simulink model "calcul_vitesse_roues"  (R2024b)
settings: Solver=FixedStepDiscrete  StartTime=0.0  StopTime=10.0  FixedStep=Ts  RelTol=1e-3
values from neighbouring files (symbols this model uses):
  J = 0.5    [main_data_vehicle.m]
  Re = 0.228    [main_data_vehicle.m]
  v0 = 0.1    [main_data_vehicle.m]
undefined symbols (not defined in the file or in its folder): DiscIntNeverNeededParam
settings Model: Creator=marti  LastModifiedBy=marti

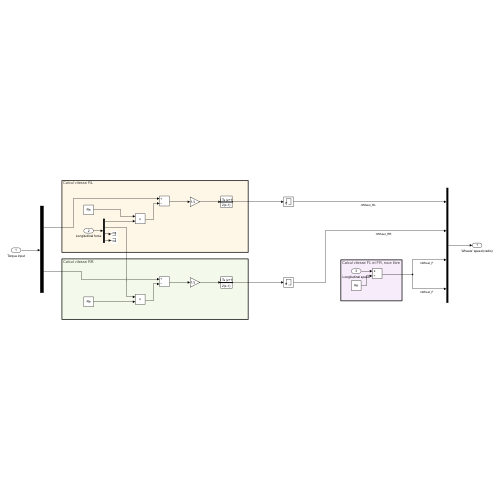
[thumbnail: Simulink's stored preview of the top-level diagram]
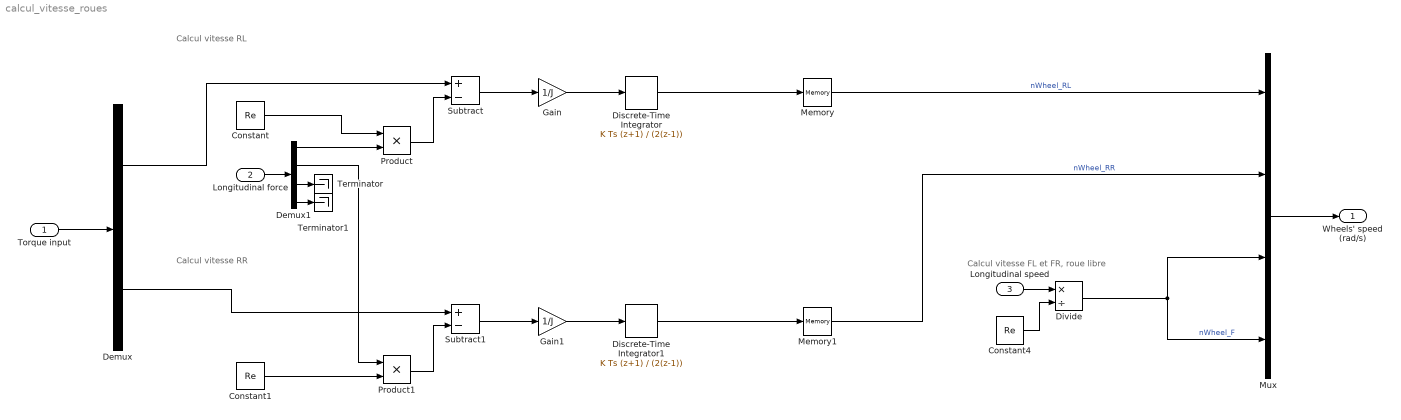
== system calcul_vitesse_roues ==
  note: Calcul vitesse FL et FR, roue libre
  note: Calcul vitesse RL
  note: Calcul vitesse RR
  Torque input : Inport
  Longitudinal force : Inport  Port=2
  Longitudinal speed : Inport  Port=3
  Constant : Constant  Value=Re
  Constant1 : Constant  Value=Re
  Constant4 : Constant  Value=Re
  Demux : Demux  Outputs=2
  Demux1 : Demux
  Discrete-Time Integrator : DiscreteIntegrator  IntegratorMethod=Integration: Trapezoidal  InitialCondition=v0/Re  SampleTime=-1  ICPrevOutput=DiscIntNeverNeededParam  ICPrevScaledInput=DiscIntNeverNeededParam
  Discrete-Time Integrator1 : DiscreteIntegrator  IntegratorMethod=Integration: Trapezoidal  InitialCondition=v0/Re  SampleTime=-1  ICPrevOutput=DiscIntNeverNeededParam  ICPrevScaledInput=DiscIntNeverNeededParam
  Divide : Product  Inputs=*/
  Gain : Gain  Gain=1/J
  Gain1 : Gain  Gain=1/J
  Memory : Memory  InitialCondition=v0/Re
  Memory1 : Memory  InitialCondition=v0/Re
  Mux : Mux
  Product : Product
  Product1 : Product
  Subtract : Sum  Inputs=+-
  Subtract1 : Sum  Inputs=+-
  Terminator : Terminator
  Terminator1 : Terminator
  Wheels' speed (rad/s) : Outport
  wires:
  Product/1 -> Subtract/2
  Subtract/1 -> Gain/1
  Torque input/1 -> Demux/1
  Demux/1 -> Subtract/1
  Longitudinal speed/1 -> Divide/1
  Constant4/1 -> Divide/2
  Mux/1 -> Wheels' speed (rad/s)/1
  Longitudinal force/1 -> Demux1/1
  Demux1/1 -> Product/2
  Constant/1 -> Product/1
  Gain/1 -> Discrete-Time Integrator/1
  Product1/1 -> Subtract1/2
  Gain1/1 -> Discrete-Time Integrator1/1
  Subtract1/1 -> Gain1/1
  Constant1/1 -> Product1/2
  Demux1/2 -> Product1/1
  Demux/2 -> Subtract1/1
  Demux1/3 -> Terminator/1
  Demux1/4 -> Terminator1/1
  Discrete-Time Integrator/1 -> Memory/1
  Discrete-Time Integrator1/1 -> Memory1/1
  Divide/1 -> Mux/3, Mux/4  "nWheel_F"
  Memory/1 -> Mux/1  "nWheel_RL"
  Memory1/1 -> Mux/2  "nWheel_RR"
